simulink subsystem "LQR"  (R2026a)
settings: Solver=VariableStepAuto
settings Model: Creator=maxim  LastModifiedBy=maxim

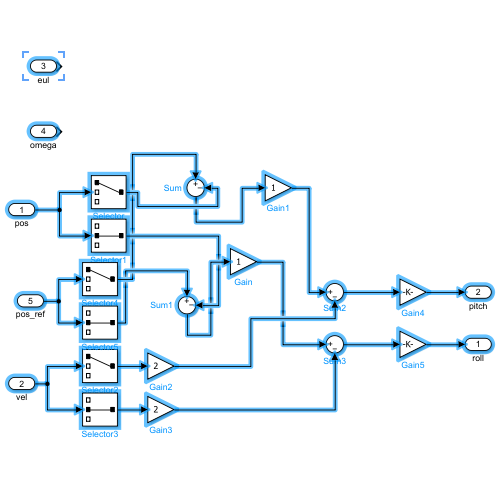
[thumbnail: Simulink's stored preview of the top-level diagram]
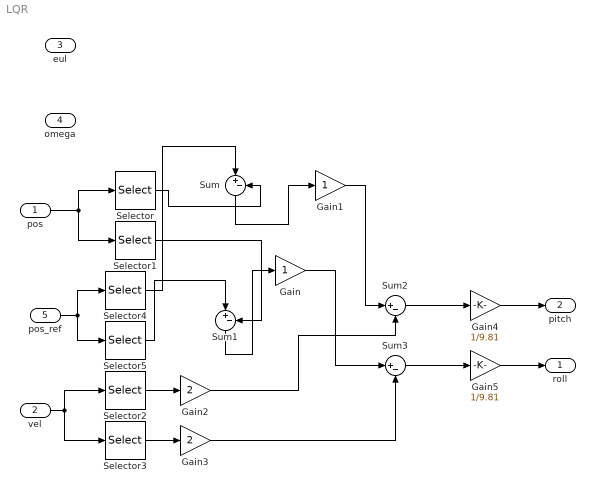
== system LQR ==
  pos : Inport
  vel : Inport  Port=2
  eul : Inport  Port=3
  omega : Inport  Port=4
  pos_ref : Inport  Port=5
  Gain : Gain
  Gain1 : Gain
  Gain2 : Gain  Gain=2
  Gain3 : Gain  Gain=2
  Gain4 : Gain  Gain=1/9.81
  Gain5 : Gain  Gain=1/9.81
  Selector : Selector  InputPortWidth=3  IndexOptions=Index vector (dialog)  Indices=1  OutputSizes=1
  Selector1 : Selector  InputPortWidth=3  IndexOptions=Index vector (dialog)  Indices=2  OutputSizes=1
  Selector2 : Selector  InputPortWidth=3  IndexOptions=Index vector (dialog)  Indices=1  OutputSizes=1
  Selector3 : Selector  InputPortWidth=3  IndexOptions=Index vector (dialog)  Indices=2  OutputSizes=1
  Selector4 : Selector  InputPortWidth=3  IndexOptions=Index vector (dialog)  Indices=1  OutputSizes=1
  Selector5 : Selector  InputPortWidth=3  IndexOptions=Index vector (dialog)  Indices=2  OutputSizes=1
  Sum{,1..3} (4 alike) : Sum  Inputs=|+-
  roll : Outport
  pitch : Outport  Port=2
  wires:
  pos/1 -> Selector1/1, Selector/1
  vel/1 -> Selector2/1, Selector3/1
  pos_ref/1 -> Selector5/1, Selector4/1
  Selector4/1 -> Sum/1
  Selector/1 -> Sum/2
  Selector5/1 -> Sum1/1
  Selector1/1 -> Sum1/2
  Sum1/1 -> Gain/1
  Sum/1 -> Gain1/1
  Selector3/1 -> Gain3/1
  Selector2/1 -> Gain2/1
  Gain1/1 -> Sum2/1
  Gain2/1 -> Sum2/2
  Gain/1 -> Sum3/1
  Gain3/1 -> Sum3/2
  Gain4/1 -> pitch/1
  Gain5/1 -> roll/1
  Sum3/1 -> Gain5/1
  Sum2/1 -> Gain4/1
